simulink model "three_phase_Kalman_fil"  (R2018a)
settings: Solver=VariableStepAuto  StartTime=0.0  StopTime=5  RelTol=1e-3
values from neighbouring files (symbols this model uses):
  k1 = K(1)    [Three_phase_Kalman_Parameter.m]
  k2 = K(2)    [Three_phase_Kalman_Parameter.m]
  Ts = dt    (= 0.01)    [Parameter.m]    (also in Three_phase_Kalman_Parameter.m = 0.0001)
libraries: powerlib_meascontrol x3
settings Model: Creator=User  LastModifiedBy=User
settings DebuggingCC: AlgebraicLoopMsg=none

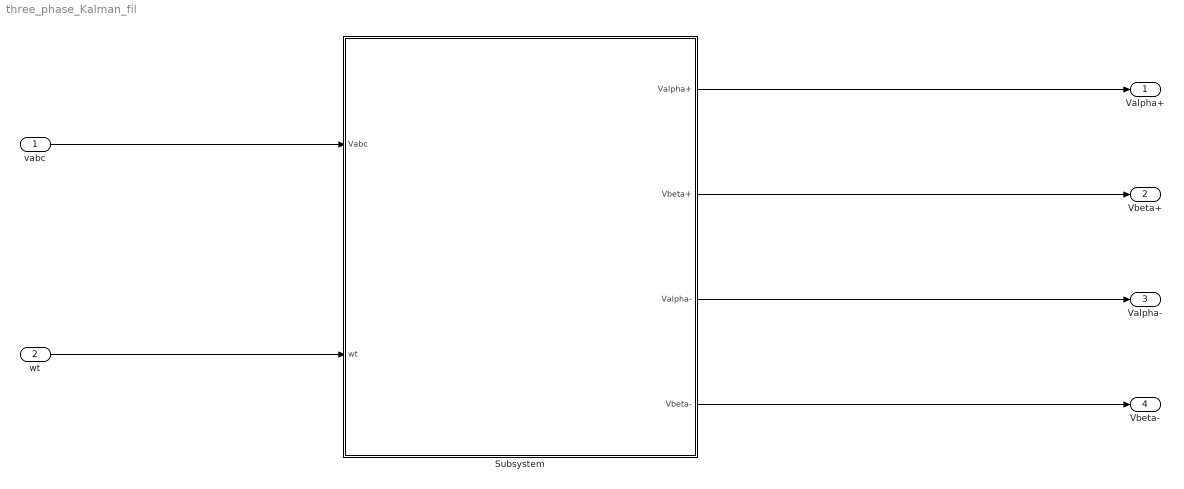
== system three_phase_Kalman_fil ==
  vabc : Inport
  wt : Inport  Port=2
  Subsystem : Subsystem
  Valpha+ : Outport
  Vbeta+ : Outport  Port=2
  Valpha- : Outport  Port=3
  Vbeta- : Outport  Port=4
  wires:
  vabc/1 -> Subsystem/1(Vabc)
  wt/1 -> Subsystem/2(wt)
  Subsystem/1(Valpha+) -> Valpha+/1
  Subsystem/2(Vbeta+) -> Vbeta+/1
  Subsystem/3(Valpha-) -> Valpha-/1
  Subsystem/4(Vbeta-) -> Vbeta-/1

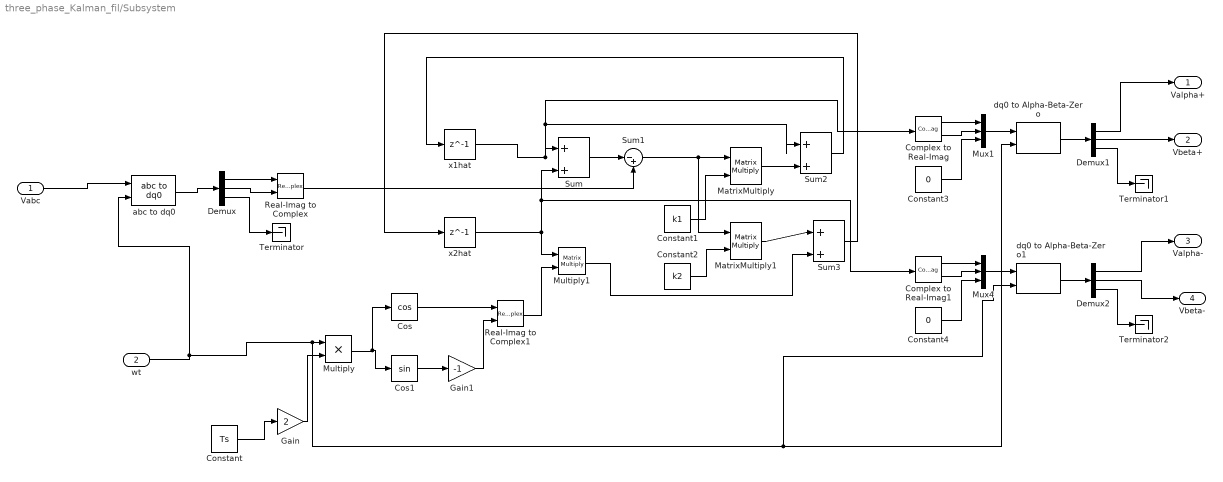
== system three_phase_Kalman_fil/Subsystem ==
  Vabc : Inport
  wt : Inport  Port=2
  Complex to Real-Imag : ComplexToRealImag
  Complex to Real-Imag1 : ComplexToRealImag
  Constant : Constant  Value=Ts
  Constant1 : Constant  Value=k1
  Constant2 : Constant  Value=k2
  Constant3 : Constant  Value=0
  Constant4 : Constant  Value=0
  Cos : Trigonometry  Operator=cos
  Cos1 : Trigonometry
  Demux : Demux  Outputs=3
  Demux1 : Demux  Outputs=3
  Demux2 : Demux  Outputs=3
  Gain : Gain  Gain=2
  Gain1 : Gain  Gain=-1
  MatrixMultiply : Product  Multiplication=Matrix(*)
  MatrixMultiply1 : Product  Multiplication=Matrix(*)
  Multiply : Product
  Multiply1 : Product  Multiplication=Matrix(*)
  Mux1 : Mux  Inputs=3
  Mux4 : Mux  Inputs=3
  Real-Imag to Complex : RealImagToComplex
  Real-Imag to Complex1 : RealImagToComplex
  Sum : Sum  Inputs=|++
  Sum1 : Sum  Inputs=|-+
  Sum2 : Sum  Inputs=|++
  Sum3 : Sum  Inputs=|++
  Terminator : Terminator
  Terminator1 : Terminator
  Terminator2 : Terminator
  abc to dq0 : powerlib_meascontrol/Transformations/abc to dq0  Alignment=90 degrees behind phase A axis
  dq0 to Alpha-Beta-Zero : powerlib_meascontrol/Transformations/dq0 to Alpha-Beta-Zero  Alignment=90 degrees behind phase A axis
      settings: SourceProductName=Simscape Power Systems  SourceProductBaseCode=PS
  dq0 to Alpha-Beta-Zero1 : powerlib_meascontrol/Transformations/dq0 to Alpha-Beta-Zero  Alignment=90 degrees behind phase A axis
      settings: SourceProductName=Simscape Power Systems  SourceProductBaseCode=PS
  x1hat : Delay  DelayLength=1  SampleTime=Ts
  x2hat : Delay  DelayLength=1  SampleTime=Ts
  Valpha+ : Outport
  Vbeta+ : Outport  Port=2
  Valpha- : Outport  Port=3
  Vbeta- : Outport  Port=4
  wires:
  Cos/1 -> Real-Imag to Complex1/1
  wt/1 -> abc to dq0/2, dq0 to Alpha-Beta-Zero1/2, dq0 to Alpha-Beta-Zero/2, Multiply/1
  Constant1/1 -> MatrixMultiply/2
  Constant/1 -> Gain/1
  x2hat/1 -> Sum/2, Complex to Real-Imag1/1, Multiply1/1
  Constant2/1 -> MatrixMultiply1/2
  Gain1/1 -> Real-Imag to Complex1/2
  Cos1/1 -> Gain1/1
  Demux/1 -> Real-Imag to Complex/1
  Complex to Real-Imag/2 -> Mux1/2
  Demux/3 -> Terminator/1
  x1hat/1 -> Sum2/1, Complex to Real-Imag/1, Sum/1
  abc to dq0/1 -> Demux/1
  Complex to Real-Imag1/1 -> Mux4/1
  Mux1/1 -> dq0 to Alpha-Beta-Zero/1
  Demux1/1 -> Valpha+/1
  Sum/1 -> Sum1/1
  Multiply1/1 -> Sum3/2
  Sum1/1 -> MatrixMultiply1/1, MatrixMultiply/1
  Constant3/1 -> Mux1/3
  Demux1/3 -> Terminator1/1
  Real-Imag to Complex1/1 -> Multiply1/2
  Multiply/1 -> Cos1/1, Cos/1
  Constant4/1 -> Mux4/3
  dq0 to Alpha-Beta-Zero/1 -> Demux1/1
  Gain/1 -> Multiply/2
  MatrixMultiply/1 -> Sum2/2
  Sum3/1 -> x2hat/1
  dq0 to Alpha-Beta-Zero1/1 -> Demux2/1
  MatrixMultiply1/1 -> Sum3/1
  Real-Imag to Complex/1 -> Sum1/2
  Complex to Real-Imag/1 -> Mux1/1
  Mux4/1 -> dq0 to Alpha-Beta-Zero1/1
  Demux/2 -> Real-Imag to Complex/2
  Sum2/1 -> x1hat/1
  Demux2/3 -> Terminator2/1
  Demux2/2 -> Vbeta-/1
  Complex to Real-Imag1/2 -> Mux4/2
  Vabc/1 -> abc to dq0/1
  Demux2/1 -> Valpha-/1
  Demux1/2 -> Vbeta+/1
